simulink model "springdamper"  (R2022b)
settings: Solver=VariableStepAuto  StartTime=0.0  StopTime=stoptime  RelTol=1e-3
values from neighbouring files (symbols this model uses):
  c = 1    [springdamper_main.m]
  k = 1    [springdamper_main.m]
  m = 1    [springdamper_main.m]
  omega = 1    [springdamper_main.m]
  x0 = 0.5    [springdamper_main.m]
  x_p0 = 0.5    [springdamper_main.m]
settings Model: Creator=a1pab  LastModifiedBy=a1pab

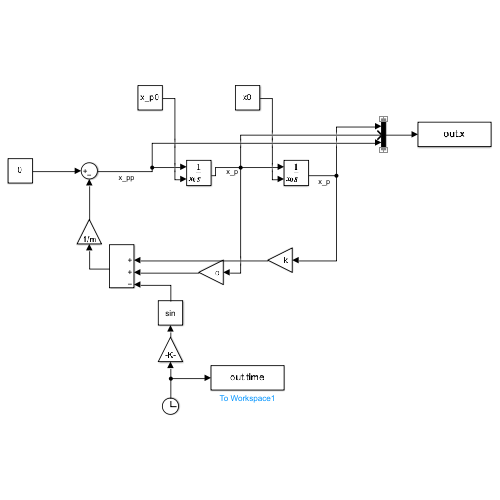
[thumbnail: Simulink's stored preview of the top-level diagram]
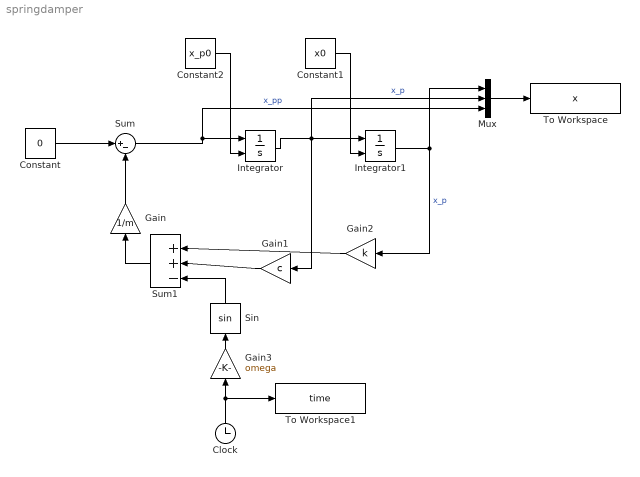
== system springdamper ==
  Clock : Clock
  Constant : Constant  Value=0
  Constant1 : Constant  Value=x0
  Constant2 : Constant  Value=x_p0
  Gain : Gain  Gain=1/m
  Gain1 : Gain  Gain=c
  Gain2 : Gain  Gain=k
  Gain3 : Gain  Gain=omega
  Integrator : Integrator  InitialConditionSource=external
  Integrator1 : Integrator  InitialConditionSource=external
  Mux : Mux  Inputs=3
  Sin : Trigonometry
  Sum : Sum  Inputs=|+-
  Sum1 : Sum  Inputs=|++-
  To Workspace : ToWorkspace  VariableName=x  SampleTime=-1
  To Workspace1 : ToWorkspace  VariableName=time  SampleTime=-1
  wires:
  Constant/1 -> Sum/1
  Integrator/1 -> Mux/2, Gain1/1, Integrator1/1  "x_p"
  Sum/1 -> Mux/3, Integrator/1  "x_pp"
  Clock/1 -> Gain3/1, To Workspace1/1
  Gain/1 -> Sum/2
  Sum1/1 -> Gain/1
  Gain1/1 -> Sum1/2
  Gain2/1 -> Sum1/1
  Integrator1/1 -> Mux/1, Gain2/1  "x_p"
  Mux/1 -> To Workspace/1
  Constant1/1 -> Integrator1/2
  Constant2/1 -> Integrator/2
  Gain3/1 -> Sin/1
  Sin/1 -> Sum1/3
